simulink library "formationFlyingBlockset"  (R2015b)
settings: Solver=ode45  StartTime=0.0  StopTime=10.0  RelTol=1e-3
undefined symbols (not defined in the file): adaptive, aircraftmask_ID, aircraftmask_navigationLaw, aircraftmask_originNED_ECEF_rrm, aircraftmask_p0_NED_m, aircraftmask_phithetapsi0, aircraftmask_phithetapsi_trim, aircraftmask_pqr0, aircraftmask_uvw0, aircraftmask_wakevortexenabled, airkraftmask_displayLeader, DiscIntNeverNeededParam, Earth, fflib_degdegm2rrm, fflib_Hz2radps, fflib_rrm2degdegm, flat2lla, hinf, innerloop, Klqr, lquadr, mask_ac, mask_ID, mpc, outerloop, poleplacement, tatestos, uavsim, washout, WGS84
libraries: formationFlyingBlockset x59, aerolibtransform2 x42, simulink_extras x27, dspsrcs4 x11, aerolibutil x5, uavsimBlockset_ServoHS55 x4, uavsimBlockset_VectorNorm x3, uavsimBlockset_UAV3DVisualization x3, uavsimBlockset_AugmentWind x3, uavsimBlockset_UAV3DInterface x3, stringquartett x2, Parrot_DCAS_lib x2
(part 3 of 5)

== system formationFlyingBlockset/Attitude laws/Local rotation angle attitude control ==
  Plant : Inport  OutDataTypeStr=Bus: StateBus
  q_c : Inport  Port=2
  Attitude control Local rotation angles : Scope  NumInputPorts=2
  Bus Selector : BusSelector  OutputSignals=alpha_rad
  Bus Selector1 : BusSelector  OutputSignals=omega_b_rps
  "Compute local theta, phi, n_z" : Subsystem
  Ground1 : Ground
  Ground3 : Ground
  Hinf law theta - phi : Subsystem
  Mux : Mux
  Radians to Degrees{,1..3} (4 alike) : simulink_extras/Transformations/Radians to Degrees
  Remove operating point offset : Sum  Inputs=+-
  Scope : Scope
  Transfer Fcn : TransferFcn  Numerator=washout.num  Denominator=washout.den
  Trim AoA : Constant  Value=mask_ac.alpha_trim
  Yaw damper : Gain  Gain=uavsim.ap.control.yawdamper.K
  get r : Selector  InputPortWidth=3  IndexOptions=Index vector (dialog)  Indices=3  OutputSizes=1
  uHinf : Scope  NumInputPorts=2
  u : Outport
  wires:
  Transfer Fcn/1 -> Yaw damper/1
  get r/1 -> Transfer Fcn/1
  Bus Selector1/1 -> get r/1  "<omega_b_rps>"
  Remove operating point offset/1 -> Hinf law theta - phi/4(alpha_rad)
  Trim AoA/1 -> Remove operating point offset/2
  Bus Selector/1 -> Remove operating point offset/1  "<alpha_rad>"
  Mux/1 -> u/1
  q_c/1 -> "Compute local theta, phi, n_z"/2(q_c)
  Ground3/1 -> Hinf law theta - phi/3("theta_c, phi_c local")
  "Compute local theta, phi, n_z"/2("p, q") -> Hinf law theta - phi/2("p, q")
  "Compute local theta, phi, n_z"/1("theta, phi local") -> Hinf law theta - phi/1("theta, phi local")
  Plant/1 -> Bus Selector/1, Bus Selector1/1, "Compute local theta, phi, n_z"/1(Plant)
  Hinf law theta - phi/2(delta_e) -> Radians to Degrees3/1, Mux/2
  Radians to Degrees3/1 -> uHinf/2  "de_deg"
  Radians to Degrees2/1 -> uHinf/1  "da_deg"
  Radians to Degrees1/1 -> Attitude control Local rotation angles/2  "phi_deg"
  Radians to Degrees/1 -> Attitude control Local rotation angles/1  "theta_deg"
  Hinf law theta - phi/4(perf_phi) -> Radians to Degrees1/1
  Hinf law theta - phi/3(perf_theta) -> Radians to Degrees/1
  Hinf law theta - phi/1(delta_a) -> Mux/1, Radians to Degrees2/1
  Yaw damper/1 -> Mux/3, Scope/1
  Ground1/1 -> Mux/4

== system formationFlyingBlockset/Command laws - code generation -/LQR altitude ==
  State estimate : Inport
  Add1 : Sum  Inputs=+-
  Bus Selector2 : BusSelector  OutputSignals=p_ned_m,v_ned_mps
  Discrete-Time Integrator : DiscreteIntegrator  InitialConditionSetting=State (most efficient)  SampleTime=-1  ICPrevOutput=DiscIntNeverNeededParam  ICPrevScaledInput=DiscIntNeverNeededParam
  K LQR : Gain  Gain=lquadr.altitudeQuad.K  Multiplication=Matrix(K*u)
  Mux2 : Mux  Inputs=3
  Scope1 : Scope
  Selector : Selector  InputPortWidth=3  IndexOptions=Index vector (dialog)  Indices=3  OutputSizes=1
  Selector1 : Selector  InputPortWidth=3  IndexOptions=Index vector (dialog)  Indices=3  OutputSizes=1
  desired z_NED_m : Constant  Value=-1
  u : Outport
  wires:
  Selector/1 -> Add1/1  "z"
  Bus Selector2/1 -> Selector/1  "<p_ned_m>"
  Bus Selector2/2 -> Selector1/1  "<v_ned_mps>"
  Add1/1 -> Scope1/1, Mux2/1, Discrete-Time Integrator/1  "z"
  Selector1/1 -> Mux2/2  "vz"
  Discrete-Time Integrator/1 -> Mux2/3
  Mux2/1 -> K LQR/1
  K LQR/1 -> u/1
  desired z_NED_m/1 -> Add1/2
  State estimate/1 -> Bus Selector2/1

== system formationFlyingBlockset/Command laws - code generation -/LQR attitude ==
  State estimate : Inport
  Bus Selector1 : BusSelector  OutputSignals=quat_be,omega_b_rps
  Discrete-Time Integrator1 : DiscreteIntegrator  InitialConditionSetting=State (most efficient)  SampleTime=-1  ICPrevOutput=DiscIntNeverNeededParam  ICPrevScaledInput=DiscIntNeverNeededParam
  K LQR1 : Gain  Gain=lquadr.attitudeQuad.K  Multiplication=Matrix(K*u)
  Mux : Mux  Inputs=2
  Mux1 : Mux  Inputs=2
  Quaternions to Rotation Angles : aerolibtransform2/Quaternions to Rotation Angles  rotationOrder=ZYX
  Scope : Scope
  u : Outport
  wires:
  Quaternions to Rotation Angles/1 -> Mux/1, Discrete-Time Integrator1/1
  Mux/1 -> Mux1/1
  K LQR1/1 -> Scope/1, u/1
  Discrete-Time Integrator1/1 -> Mux1/2
  Mux1/1 -> K LQR1/1
  State estimate/1 -> Bus Selector1/1
  Bus Selector1/1 -> Quaternions to Rotation Angles/1  "<quat_be>"
  Bus Selector1/2 -> Mux/2  "<omega_b_rps>"

== system formationFlyingBlockset/Command laws - code generation -/LQR roll & pitch ==
  State estimate : Inport
  Bus Selector1 : BusSelector  OutputSignals=quat_be,omega_b_rps
  Discrete-Time Integrator1 : DiscreteIntegrator  InitialConditionSetting=State (most efficient)  SampleTime=-1  ICPrevOutput=DiscIntNeverNeededParam  ICPrevScaledInput=DiscIntNeverNeededParam
  K LQR1 : Gain  Gain=lquadr.rollpitchQuad.K  Multiplication=Matrix(K*u)
  Mux : Mux  Inputs=2
  Mux1 : Mux  Inputs=2
  Quaternions to Rotation Angles : aerolibtransform2/Quaternions to Rotation Angles  rotationOrder=ZYX
  "get p, q" : Selector  InputPortWidth=3  IndexOptions=Index vector (dialog)  Indices=[1 2]  OutputSizes=1
  "get theta, phi" : Selector  InputPortWidth=3  IndexOptions=Index vector (dialog)  Indices=[2 3]  OutputSizes=1
  u : Outport
  wires:
  Bus Selector1/2 -> "get p, q"/1  "<omega_b_rps>"
  Quaternions to Rotation Angles/1 -> "get theta, phi"/1
  Bus Selector1/1 -> Quaternions to Rotation Angles/1  "<quat_be>"
  "get p, q"/1 -> Mux/2
  State estimate/1 -> Bus Selector1/1
  Mux1/1 -> K LQR1/1
  Discrete-Time Integrator1/1 -> Mux1/2
  K LQR1/1 -> u/1
  Mux/1 -> Mux1/1
  "get theta, phi"/1 -> Discrete-Time Integrator1/1, Mux/1

== system formationFlyingBlockset/Cularis/Wake vortex effects ==
  AirframeBus : Inport  OutDataTypeStr=Bus: Airframe
  Environment : Inport  Port=2  OutDataTypeStr=Bus: Environment
  Ci_w : Inport  Port=3
  Augment atmospheric wind and wind gradients by induced wind and effects of induced wind gradients : uavsimBlockset_AugmentWind/Augment atmospheric wind and wind gradients by induced wind and induced wind gradients
  Constant : Constant  Value=aircraftmask_wakevortexenabled
  Constant1 : Constant  Value=zeros(3,1)
  Constant2 : Constant  Value=zeros(3,1)
  If : If  IfExpression=u1 ~= 0
  Subsystem : Subsystem
  Switch : Switch  Criteria=u2 ~= 0
  Switch1 : Switch  Criteria=u2 ~= 0
  Terminator : Terminator
  EnvData_augmented : Outport  OutDataTypeStr=Bus: Environment
  Vi_bfrozen : Outport  Port=2
  wires:
  AirframeBus/1 -> Subsystem/1(AirframeBus)
  Constant/1 -> Switch/2, Switch1/2, If/1
  Ci_w/1 -> Subsystem/2(Ci_w)
  Environment/1 -> Augment atmospheric wind and wind gradients by induced wind and effects of induced wind gradients/1
  Subsystem/1(Vi_bfrozen) -> Switch/1
  Subsystem/2(omegai_bfrozen) -> Switch1/1
  Constant1/1 -> Switch/3
  Switch/1 -> Vi_bfrozen/1, Augment atmospheric wind and wind gradients by induced wind and effects of induced wind gradients/2
  Switch1/1 -> Augment atmospheric wind and wind gradients by induced wind and effects of induced wind gradients/3
  Constant2/1 -> Switch1/3
  Augment atmospheric wind and wind gradients by induced wind and effects of induced wind gradients/1 -> EnvData_augmented/1
  If/1 -> Subsystem/Action
  If/2 -> Terminator/1

== system formationFlyingBlockset/Fixed wing avionics/Command laws ==
  Aircraft state estimate : Inport  OutDataTypeStr=Bus: StateBus
  iUASCom : Inport  Port=2  OutDataTypeStr=Bus: iUAScom
  formationOffset_m : Inport  Port=3
  fstate_dx_in : Inport  Port=4
  vLeaderState : Inport  Port=5  OutDataTypeStr=Bus: iUAScom
  Add1 : Sum
  Adds Separate Surface Excitations for system identification : Subsystem
  Constant : Constant  Value=100
  Constant1 : Constant  Value=aircraftmask_ID
  Constant2 : Constant  Value=airkraftmask_displayLeader
  Control laws : Subsystem  SystemSampleTime=uavsim.ap.hardware.dt_navigationloops_s
  If : If  IfExpression=u1 ~= 0  SampleTime=uavsim.ap.hardware.dt_navigationloops_s
  Leader NED position : formationFlyingBlockset/Signal to workspace  mask_id=['log_pNED_leader_UAS' num2str(aircraftmask_ID) ]  mask_dt=0.1  mask_debug=log_pNED_leader_UAS1
  Leader NED velocity : formationFlyingBlockset/Signal to workspace  mask_id=['log_vNED_leader_UAS' num2str(aircraftmask_ID) ]  mask_dt=0.1  mask_debug=log_vNED_leader_UAS1
  Scope : Scope
  Subsystem : Subsystem
  Terminator : Terminator
  u - system inputs : Outport  OutDataTypeStr=Bus: CMD
  fstate_dx : Outport  Port=2
  wires:
  Add1/1 -> Subsystem/1(In1)
  vLeaderState/1 -> Control laws/5(vLeaderState)
  Constant2/1 -> If/1
  If/1 -> Subsystem/Action
  If/2 -> Terminator/1
  Aircraft state estimate/1 -> Control laws/1(Plant)
  iUASCom/1 -> Control laws/2(iUASCom)
  formationOffset_m/1 -> Control laws/3(formationOffset_m)
  Constant1/1 -> Add1/1
  Constant/1 -> Add1/2
  Control laws/2(vc_NED_mps) -> Leader NED velocity/1, Subsystem/3(In3)
  Control laws/1(pc_NED_m) -> Scope/1, Leader NED position/1, Subsystem/2(In2)
  Adds Separate Surface Excitations for system identification/1(u + SSE) -> u - system inputs/1
  Control laws/3(CMD) -> Adds Separate Surface Excitations for system identification/1(u)
  Control laws/4(fstate_dx) -> fstate_dx/1
  fstate_dx_in/1 -> Control laws/4(fstate_dx_in)

== system formationFlyingBlockset/Fixed wing avionics/Sensor delays1 ==
  sensor readings : Inport  OutDataTypeStr=Bus: SensorBus
  Bus Creator : BusCreator  Inputs=7  OutDataTypeStr=Bus: SensorBus
  Bus Selector : BusSelector  OutputSignals=ahrs,airdata,gnss_l1,gnss_rtk,propulsion,radiodistance,windangles
  estimated aircraft state : Outport  OutDataTypeStr=Bus: StateBus
  wires:
  sensor readings/1 -> Bus Selector/1
  ? -> estimated aircraft state/1

== system formationFlyingBlockset/Parrot drone open loop dynamics/Vehicle model ==
  CMD : Inport  OutDataTypeStr=Bus: CMD_quadrotor
  EnvData : Inport  Port=2
  FM_external : Inport  Port=3
  Bus Selector2 : BusSelector  OutputSignals=groundlevel_NED_m,glocal_ms2
  Bus Selector3 : BusSelector  OutputSignals=RotationalVelocity.omega_b_rps,Velocity.Vground_bfrozen_mps,Attitude.euler_rad
  FIXME Remove algebraic loop : Memory  X0=1e-6
  Kinematics : uavsimblockset_SixDOFKinematics/Aircraft kinematics  mask_inertia=Itot  mask_mass=mtot  mask_P0_ECEF_rrm=mask_p0_ECEF_lla  mask_originNED_ECEF_rrm=mask_originNED_ECEF_rrm  mask_uvw0=mask_uvw0  mask_phithetapsi0=mask_phithetapsi0  mask_omega0=mask_pqr0
  ModelBus6 : BusCreator  Inputs=2  OutDataTypeStr=Bus: Airframe  NonVirtualBus=on
  Parrot dynamics : Subsystem
  Airframe : Outport  OutDataTypeStr=Bus: Airframe
  Cwind : Outport  Port=2
  FMprop : Outport  Port=3
  wires:
  FIXME Remove algebraic loop/1 -> ModelBus6/1, Bus Selector3/1  "Kinematics"
  Bus Selector2/1 -> Kinematics/1  "<groundlevel_NED_m>"
  Bus Selector2/2 -> Kinematics/4  "<glocal_ms2>"
  Bus Selector3/1 -> Parrot dynamics/3(omega_bfrozen_rps)  "<omega_b_rps>"
  Bus Selector3/2 -> Parrot dynamics/4(Vground_bfrozen_mps)  "<Vground_bfrozen_mps>"
  ModelBus6/1 -> Airframe/1
  Parrot dynamics/2(AeroBus) -> ModelBus6/2
  EnvData/1 -> Bus Selector2/1, Parrot dynamics/2(EnvData)
  FM_external/1 -> Kinematics/3
  Parrot dynamics/3(Coefficients_windframe) -> Cwind/1
  Parrot dynamics/1(FMaero_bf) -> Kinematics/2
  Kinematics/1 -> FIXME Remove algebraic loop/1
  CMD/1 -> Parrot dynamics/1(CMD)
  Bus Selector3/3 -> Parrot dynamics/5(eulers)  "<euler_rad>"

== system formationFlyingBlockset/Quadcopter avionics/Command laws - code generation - ==
  Aircraft state estimate : Inport  OutDataTypeStr=Bus: StateBus
  Control laws : Subsystem  TreatAsAtomicUnit=on  SystemSampleTime=uavsim.ap.hardware.dt_attitudeloops_s
  u - system inputs : Outport  OutDataTypeStr=Bus: CMD
  wires:
  Control laws/1(engine commands) -> u - system inputs/1
  Aircraft state estimate/1 -> Control laws/1(Plant state estimate)

== system formationFlyingBlockset/Quadcopter avionics/Sensor delays1 ==
  sensor readings : Inport  OutDataTypeStr=Bus: SensorBus
  Bus Creator : BusCreator  Inputs=7  OutDataTypeStr=Bus: SensorBus
  Bus Selector : BusSelector  OutputSignals=ahrs,airdata,gnss_l1,gnss_rtk,propulsion,radiodistance,windangles
  estimated aircraft state : Outport  OutDataTypeStr=Bus: StateBus
  wires:
  ? -> estimated aircraft state/1
  sensor readings/1 -> Bus Selector/1

== system formationFlyingBlockset/Sensor package: error-free/AHRS ==
  aircraft state : Inport  OutDataTypeStr=Bus: Airframe
  Environment : Inport  Port=2  OutDataTypeStr=Bus: Environment
  Add gravity : Sum
  Bus Creator : BusCreator  Inputs=3  OutDataTypeStr=Bus: AHRS
  Bus Selector : BusSelector  OutputSignals=Kinematics.Attitude.DCM_be,Kinematics.RotationalVelocity.omega_b_rps,Kinematics.Acceleration.VgroundDot_bfrozen_mps2,Kinematics.RotationalAcceleration.omegaDot_b_rps2
  Bus Selector1 : BusSelector  OutputSignals=glocal_ms2
  Constant : Constant  Value=[0 0 0]'
  Constant1 : Constant  Value=[0 0]'
  Direction Cosine Matrix to Quaternions : aerolibtransform2/Direction Cosine Matrix  to Quaternions
  Mux : Mux  Inputs=2
  Mux2 : Mux  Inputs=2
  Scope1 : Scope
  Three-axis Accelerometer : aerolibnav/Three-axis Accelerometer  units=Metric (MKS)  acc=[0 0 0]  gtype=off  dtype_a=off  w_a=190  z_a=0.707  a_sf_cc=[1 0 0; 0 1 0; 0 0 1]  a_bias=[0 0 0]  a_Ts=0.01  a_rand=off  a_seeds=[23093 23094 23095]  a_pow=0.01 * [0.0101 0.0116 0.0144] .^ 2  a_sat="[-inf  -inf  -inf  inf inf inf]"
  Three-axis Gyroscope : aerolibnav/Three-axis Gyroscope  dtype_g=off  w_g=190  z_g=0.707  g_sf_cc=[1 0 0; 0 1 0; 0 0 1]  g_bias=[0 0 0]  g_sen=[0 0 0]  g_Ts=0.01  g_rand=off  g_seeds=[23093 23094 23095]  g_pow="0.01 * (1e-3 * [0.8056    0.5346    0.9000]) .^2"  g_sat="[-inf  -inf  -inf  inf inf inf]"
  gravity to body frame : Product  Multiplication=Matrix(*)
  unit conversion: mps2 to g : formationFlyingBlockset/unit conversion: mps2 to g
  output : Outport  OutDataTypeStr=Bus: AHRS
  wires:
  Mux2/1 -> Scope1/1
  Bus Creator/1 -> output/1
  aircraft state/1 -> Bus Selector/1
  Bus Selector/1 -> Direction Cosine Matrix to Quaternions/1, gravity to body frame/1  "<DCM_be>"
  Direction Cosine Matrix to Quaternions/1 -> Bus Creator/1  "quat"
  Bus Selector/2 -> Three-axis Gyroscope/1, Three-axis Accelerometer/2  "<omega_b_rps>"
  Bus Selector/3 -> Add gravity/1  "<VgroundDot_bfrozen_mps2>"
  Three-axis Gyroscope/1 -> Bus Creator/2  "gyro_rps"
  Three-axis Accelerometer/1 -> Bus Creator/3, Mux2/1  "acc_mps2"
  Bus Selector/4 -> Three-axis Accelerometer/3  "<omegaDot_b_rps2>"
  Constant/1 -> Three-axis Accelerometer/4
  Bus Selector1/1 -> Mux/2  "<glocal_ms2>"
  Environment/1 -> Bus Selector1/1
  gravity to body frame/1 -> Add gravity/2
  Constant1/1 -> Mux/1
  Mux/1 -> gravity to body frame/2
  Add gravity/1 -> unit conversion: mps2 to g/1, Three-axis Accelerometer/1, Mux2/2
  unit conversion: mps2 to g/1 -> Three-axis Gyroscope/2

== system formationFlyingBlockset/Sensor package: error-free/Air Data ==
  aircraft state : Inport  OutDataTypeStr=Bus: Airframe
  Bus Creator : BusCreator  Inputs=3  OutDataTypeStr=Bus: Airdata
  Bus Selector : BusSelector  OutputSignals=Kinematics.Position.P_LLA_deg_m,Aero.qbar_Pa
  Gain : Gain
  ISA Atmosphere Model : aerolibatmos2/ISA Atmosphere Model  custom=off  g=9.80665  gamma=1.4  R=287.0531  L=0.0065  h_trop=11000  h_strat=20000  rho0=1.225  P0=101325  T0=288.15  h0=0
  Terminator : Terminator
  Terminator1 : Terminator
  get altitude : Selector  InputPortWidth=3  IndexOptions=Index vector (dialog)  Indices=3  OutputSizes=1
  output : Outport  OutDataTypeStr=Bus: Airdata
  wires:
  get altitude/1 -> ISA Atmosphere Model/1
  Gain/1 -> Bus Creator/3  "qBar_Pa"
  ISA Atmosphere Model/4 -> Terminator1/1
  ISA Atmosphere Model/2 -> Terminator/1
  ISA Atmosphere Model/3 -> Bus Creator/2  "pStat_Pa"
  ISA Atmosphere Model/1 -> Bus Creator/1  "Tair_K"
  Bus Selector/1 -> get altitude/1  "<P_LLA_deg_m>"
  Bus Selector/2 -> Gain/1  "<qbar_Pa>"
  Bus Creator/1 -> output/1
  aircraft state/1 -> Bus Selector/1

== system formationFlyingBlockset/Sensor package: error-free/L1 GPS ==
  aircraft state : Inport  OutDataTypeStr=Bus: Airframe
  Bus Creator : BusCreator  Inputs=2  OutDataTypeStr=Bus: GNSSL1
      settings: InheritFromInputs=off
  Bus Selector1 : BusSelector  OutputSignals=Kinematics.Position.P_ECEF_m,Kinematics.Velocity.Vground_ECEF_mps
  Gain : Gain
  Gain1 : Gain
  output : Outport  OutDataTypeStr=Bus: GNSSL1
  wires:
  Gain1/1 -> Bus Creator/2  "v_ecef_m"
  Gain/1 -> Bus Creator/1  "p_ecef_m"
  Bus Selector1/2 -> Gain1/1  "<Vground_ECEF_mps>"
  Bus Selector1/1 -> Gain/1  "<P_ECEF_m>"
  Bus Creator/1 -> output/1
  aircraft state/1 -> Bus Selector1/1

== system formationFlyingBlockset/Sensor package: error-free/Optitrack ==
  aircraft state : Inport  OutDataTypeStr=Bus: Airframe
  Bus Creator : BusCreator  Inputs=2  OutDataTypeStr=Bus: MotionTracker
      settings: InheritFromInputs=off
  Bus Selector : BusSelector  OutputSignals=Kinematics.Position.P_NED_m,Kinematics.Velocity.Vground_NED_mps
  Gain : Gain
  Gain1 : Gain
  output : Outport  OutDataTypeStr=Bus: MotionTracker
  wires:
  Bus Creator/1 -> output/1
  aircraft state/1 -> Bus Selector/1
  Bus Selector/1 -> Gain/1  "<P_NED_m>"
  Gain/1 -> Bus Creator/1  "p_ned_m"
  Bus Selector/2 -> Gain1/1  "<Vground_NED_mps>"
  Gain1/1 -> Bus Creator/2  "v_ned_mps"

== system formationFlyingBlockset/Sensor package: error-free/Propulsion sensors ==
  aircraft state : Inport  OutDataTypeStr=Bus: Airframe
  Bus Creator : BusCreator  Inputs=2  OutDataTypeStr=Bus: Enginedata
      settings: InheritFromInputs=off
  I : Constant  Value=0
  U : Constant  Value=0
  output : Outport  OutDataTypeStr=Bus: Enginedata
  wires:
  Bus Creator/1 -> output/1
  I/1 -> Bus Creator/2  "I"
  U/1 -> Bus Creator/1  "U"

== system formationFlyingBlockset/Sensor package: error-free/RTK DGPS ==
  aircraft state : Inport  OutDataTypeStr=Bus: Airframe
  inter UAS com : Inport  Port=2  OutDataTypeStr=Bus: iUAScom
  Bus Creator : BusCreator  Inputs=2  OutDataTypeStr=Bus: GNSSRTK
      settings: InheritFromInputs=off
  Bus Selector : BusSelector  OutputSignals=P_NED_m,Vground_NED_mps
  Bus Selector1 : BusSelector  OutputSignals=Kinematics.Position.P_NED_m,Kinematics.Velocity.Vground_NED_mps
  Delta position : Sum  Inputs=+-
  Delta velocity : Sum  Inputs=+-
  Flat Earth to LLA{,2..4} (4 alike) : aerolibtransform2/Flat Earth to LLA  units=Metric (MKS)  ptype=Earth (WGS84)  F=1/298.257223563  R=6378137  LL0=rad2deg(aircraftmask_originNED_ECEF_rrm(1:2))  psi=0
  LLA to ECEF Position{,2..4} (4 alike) : aerolibtransform2/LLA to ECEF Position  units=Metric (MKS)  ptype=Earth (WGS84)  F=1/298.257223563  R=6378137
  Scope : Scope
  Scope1 : Scope
  Scope2 : Scope
  href NED : Constant  Value=aircraftmask_originNED_ECEF_rrm(3)
  output : Outport  OutDataTypeStr=Bus: GNSSRTK
  wires:
  Delta velocity/1 -> Bus Creator/2  "delta_v_ecef_mps"
  LLA to ECEF Position3/1 -> Delta velocity/1
  LLA to ECEF Position4/1 -> Delta velocity/2
  Flat Earth to LLA4/1 -> LLA to ECEF Position4/1
  Flat Earth to LLA4/2 -> LLA to ECEF Position4/2
  Bus Selector/2 -> Flat Earth to LLA4/1  "<Vground_NED_mps>"
  Flat Earth to LLA3/1 -> LLA to ECEF Position3/1
  Flat Earth to LLA3/2 -> LLA to ECEF Position3/2
  href NED/1 -> Flat Earth to LLA/2, Flat Earth to LLA2/2, Flat Earth to LLA4/2, Flat Earth to LLA3/2
  Bus Selector1/2 -> Flat Earth to LLA3/1  "<Vground_NED_mps>"
  LLA to ECEF Position/1 -> Delta position/1
  LLA to ECEF Position2/1 -> Delta position/2
  Flat Earth to LLA2/1 -> LLA to ECEF Position2/1
  Flat Earth to LLA2/2 -> LLA to ECEF Position2/2
  Delta position/1 -> Bus Creator/1, Scope/1  "delta_p_ecef_m"
  Bus Selector/1 -> Scope2/1, Flat Earth to LLA2/1  "<P_NED_m>"
  Flat Earth to LLA/1 -> LLA to ECEF Position/1
  Flat Earth to LLA/2 -> LLA to ECEF Position/2
  Bus Selector1/1 -> Scope1/1, Flat Earth to LLA/1  "<P_NED_m>"
  Bus Creator/1 -> output/1
  aircraft state/1 -> Bus Selector1/1
  inter UAS com/1 -> Bus Selector/1

== system formationFlyingBlockset/Sensor package: error-free/Radio distance sensor ==
  aircraft state : Inport  OutDataTypeStr=Bus: Airframe
  inter UAS com : Inport  Port=2  OutDataTypeStr=Bus: iUAScom
  Bus Creator : BusCreator  Inputs=1  OutDataTypeStr=Bus: Radiodistance
      settings: InheritFromInputs=off
  Bus Selector : BusSelector  OutputSignals=P_NED_m
  Bus Selector1 : BusSelector  OutputSignals=Kinematics.Position.P_NED_m
  Delta position : Sum  Inputs=-+
  vector norm : uavsimBlockset_VectorNorm/vector norm
  output : Outport  OutDataTypeStr=Bus: Radiodistance
  wires:
  vector norm/1 -> Bus Creator/1  "r"
  Delta position/1 -> vector norm/1
  Bus Creator/1 -> output/1
  Bus Selector/1 -> Delta position/2  "<P_NED_m>"
  Bus Selector1/1 -> Delta position/1  "<P_NED_m>"
  aircraft state/1 -> Bus Selector1/1
  inter UAS com/1 -> Bus Selector/1

== system formationFlyingBlockset/Sensor package: error-free/Wind angle sensors ==
  aircraft state : Inport  OutDataTypeStr=Bus: Airframe
  Bus Creator : BusCreator  Inputs=2  OutDataTypeStr=Bus: WindAngles
  Bus Selector : BusSelector  OutputSignals=Aero.alpha_rad,Aero.beta_rad
  Gain : Gain
  Gain1 : Gain
  output : Outport  OutDataTypeStr=Bus: WindAngles
  wires:
  Gain1/1 -> Bus Creator/2  "beta_rad"
  Gain/1 -> Bus Creator/1  "alpha_rad"
  Bus Selector/2 -> Gain1/1  "<beta_rad>"
  Bus Selector/1 -> Gain/1  "<alpha_rad>"
  aircraft state/1 -> Bus Selector/1
  Bus Creator/1 -> output/1

== system formationFlyingBlockset/Wake vortex effects/Subsystem ==
  AirframeBus : Inport  OutDataTypeStr=Bus: Airframe
  Ci_w : Inport  Port=2
  Action Port : ActionPort
  Bus Selector : BusSelector  OutputSignals=Kinematics.Position.P_NED_m,Kinematics.Velocity.Vground_NED_mps,Kinematics.Attitude.DCM_be,Aero.alpha_rad,Aero.beta_rad
  Cularis Vortex model : formationFlyingBlockset/Cularis Vortex model  mask_ID=aircraftmask_ID
  Demux : Demux  Outputs=2
  Direction Cosine Matrix  to Quaternions : aerolibtransform2/Direction Cosine Matrix  to Quaternions
  Get CL : Selector  InputPortWidth=6  IndexOptions=Index vector (dialog)  Indices=3  OutputSizes=1
  Memory : Memory  X0=[0 0]
  Memory1 : Memory  X0=eye(3)
  Memory2 : Memory  X0=zeros(3,1)
  Memory3 : Memory  X0=zeros(3,1)
  Memory4 : Memory  X0=1
  Mux : Mux  Inputs=2
  Signal Conversion : SignalConversion
  Vi_bfrozen : Outport
  omegai_bfrozen : Outport  Port=2
  vortex parameters : Outport  Port=3
  wires:
  Demux/1 -> Cularis Vortex model/5
  Demux/2 -> Cularis Vortex model/6
  AirframeBus/1 -> Bus Selector/1
  Ci_w/1 -> Get CL/1
  Get CL/1 -> Memory4/1
  Direction Cosine Matrix  to Quaternions/1 -> Cularis Vortex model/4
  Bus Selector/1 -> Memory3/1  "<P_NED_m>"
  Bus Selector/2 -> Memory2/1  "<Vground_NED_mps>"
  Bus Selector/3 -> Memory1/1  "<DCM_be>"
  Bus Selector/4 -> Mux/1  "<alpha_rad>"
  Bus Selector/5 -> Mux/2  "<beta_rad>"
  Mux/1 -> Memory/1
  Memory/1 -> Demux/1
  Memory1/1 -> Direction Cosine Matrix  to Quaternions/1
  Memory2/1 -> Cularis Vortex model/2
  Memory3/1 -> Cularis Vortex model/1
  Memory4/1 -> Cularis Vortex model/3
  Cularis Vortex model/1 -> Vi_bfrozen/1
  Cularis Vortex model/2 -> omegai_bfrozen/1
  Cularis Vortex model/4 -> Signal Conversion/1
  Signal Conversion/1 -> vortex parameters/1

== system formationFlyingBlockset/Wake vortex effects/Visualize vortices in UAV3D ==
  vortex parameters : Inport
  enable UAV3D : Inport  Port=2
  Bus Selector : BusSelector  OutputSignals=p0_filament_left,p0_filament_right,dcm_ew
  Constant1 : Constant  Value=aircraftmask_ID+30
  Constant11 : Constant  Value=0.5
  Constant12 : Constant  Value=3*uavsim.cularis.b
  Constant13 : Constant  Value=0.3
  Constant2 : Constant  Value=aircraftmask_ID+60
  Display : Display
  Visualize vortex tunnel in UAV3D1 : formationFlyingBlockset/Visualize vortex tunnel in UAV3D
  Visualize vortex tunnel in UAV3D2 : formationFlyingBlockset/Visualize vortex tunnel in UAV3D
  wires:
  Bus Selector/2 -> Visualize vortex tunnel in UAV3D1/2  "<p0_filament_right>"
  Constant12/1 -> Visualize vortex tunnel in UAV3D1/4, Visualize vortex tunnel in UAV3D2/4
  Constant11/1 -> Visualize vortex tunnel in UAV3D1/3, Visualize vortex tunnel in UAV3D2/3
  Constant2/1 -> Visualize vortex tunnel in UAV3D2/1
  Bus Selector/1 -> Visualize vortex tunnel in UAV3D2/2, Display/1  "<p0_filament_left>"
  Constant1/1 -> Visualize vortex tunnel in UAV3D1/1
  Constant13/1 -> Visualize vortex tunnel in UAV3D1/5, Visualize vortex tunnel in UAV3D2/5
  vortex parameters/1 -> Bus Selector/1
  Bus Selector/3 -> Visualize vortex tunnel in UAV3D1/6, Visualize vortex tunnel in UAV3D2/6  "<dcm_ew>"
  enable UAV3D/1 -> Visualize vortex tunnel in UAV3D1/7, Visualize vortex tunnel in UAV3D2/7

== system formationFlyingBlockset/Zagi/Wake vortex effects ==
  AirframeBus : Inport  OutDataTypeStr=Bus: Airframe
  Environment : Inport  Port=2  OutDataTypeStr=Bus: Environment
  Ci_w : Inport  Port=3
  Augment atmospheric wind and wind gradients by induced wind and effects of induced wind gradients : uavsimBlockset_AugmentWind/Augment atmospheric wind and wind gradients by induced wind and induced wind gradients
  Constant : Constant  Value=aircraftmask_wakevortexenabled
  Constant1 : Constant  Value=zeros(3,1)
  Constant2 : Constant  Value=zeros(3,1)
  If : If  IfExpression=u1 ~= 0
  Subsystem : Subsystem
  Switch : Switch  Criteria=u2 ~= 0
  Switch1 : Switch  Criteria=u2 ~= 0
  Terminator : Terminator
  EnvData_augmented : Outport  OutDataTypeStr=Bus: Environment
  Vi_bfrozen : Outport  Port=2
  wires:
  AirframeBus/1 -> Subsystem/1(AirframeBus)
  Constant/1 -> Switch/2, Switch1/2, If/1
  Ci_w/1 -> Subsystem/2(Ci_w)
  Environment/1 -> Augment atmospheric wind and wind gradients by induced wind and effects of induced wind gradients/1
  Subsystem/1(Vi_bfrozen) -> Switch/1
  Subsystem/2(omegai_bfrozen) -> Switch1/1
  Constant1/1 -> Switch/3
  Switch/1 -> Vi_bfrozen/1, Augment atmospheric wind and wind gradients by induced wind and effects of induced wind gradients/2
  Switch1/1 -> Augment atmospheric wind and wind gradients by induced wind and effects of induced wind gradients/3
  Constant2/1 -> Switch1/3
  Augment atmospheric wind and wind gradients by induced wind and effects of induced wind gradients/1 -> EnvData_augmented/1
  If/1 -> Subsystem/Action
  If/2 -> Terminator/1

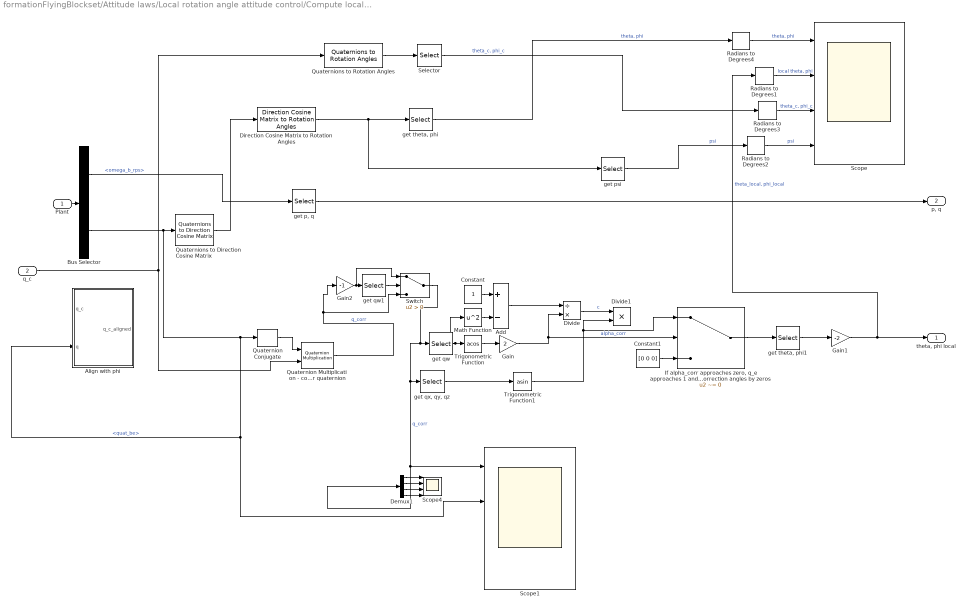
== system formationFlyingBlockset/Attitude laws/Local rotation angle attitude control/Compute local theta, phi, n_z ==
  Plant : Inport  OutDataTypeStr=Bus: StateBus
  q_c : Inport  Port=2
  Add : Sum  Inputs=+-
  Align with phi : Subsystem
  Bus Selector : BusSelector  OutputSignals=omega_b_rps,quat_be
  Constant : Constant
  Constant1 : Constant  Value=[0 0 0]
  Demux1 : Demux
  Direction Cosine Matrix to Rotation Angles : aerolibtransform2/Direction Cosine Matrix to Rotation Angles  rotationOrder=ZYX  lim=Default
      settings: AttributesFormatString=Rotation Order: %<rotationOrder>
  Divide : Product  Inputs=/*
  Divide1 : Product  Inputs=**
  Gain : Gain  Gain=2
  Gain1 : Gain  Gain=-2
  Gain2 : Gain  Gain=-1
  "If alpha_corr approaches zero, q_e approaches 1 and c goes to infinity. In that case, just replace the computed correction angles by zeros" : Switch  Criteria=u2 ~= 0
  Math Function : Math  Operator=square  SaturateOnIntegerOverflow=on
  Quaternion Conjugate : aerolibutil/Quaternion Conjugate
  Quaternion Multiplication - compute error quaternion : aerolibutil/Quaternion Multiplication
  Quaternions to Direction Cosine Matrix : aerolibtransform2/Quaternions to  Direction Cosine Matrix
  Quaternions to Rotation Angles : aerolibtransform2/Quaternions to Rotation Angles  rotationOrder=ZYX
  Radians to Degrees{1..4} (4 alike) : simulink_extras/Transformations/Radians to Degrees
  Scope : Scope  NumInputPorts=4
  Scope1 : Scope  NumInputPorts=4
  Scope4 : Scope  NumInputPorts=4
  Selector : Selector  InputPortWidth=3  IndexOptions=Index vector (dialog)  Indices=[2 3]  OutputSizes=1
  Switch : Switch  Criteria=u2 > Threshold
  Trigonometric Function : Trigonometry  Operator=acos
  Trigonometric Function1 : Trigonometry  Operator=asin
  "get p, q" : Selector  InputPortWidth=3  IndexOptions=Index vector (dialog)  Indices=[1 2]  OutputSizes=1
  get psi : Selector  InputPortWidth=3  IndexOptions=Index vector (dialog)  Indices=1  OutputSizes=1
  get qw : Selector  InputPortWidth=4  IndexOptions=Index vector (dialog)  Indices=1  OutputSizes=1
  get qw1 : Selector  InputPortWidth=4  IndexOptions=Index vector (dialog)  Indices=1  OutputSizes=1
  "get qx, qy, qz" : Selector  InputPortWidth=4  IndexOptions=Index vector (dialog)  Indices=2:4  OutputSizes=1
  "get theta, phi" : Selector  InputPortWidth=3  IndexOptions=Index vector (dialog)  Indices=[2 3]  OutputSizes=1
  "get theta, phi1" : Selector  InputPortWidth=3  IndexOptions=Index vector (dialog)  Indices=[2 1]  OutputSizes=1
  "theta, phi local" : Outport
  "p, q" : Outport  Port=2
  wires:
  get qw1/1 -> Switch/2
  Gain2/1 -> get qw1/1, Switch/1
  Quaternion Multiplication - compute error quaternion/1 -> Switch/3, Gain2/1  "q_corr"
  Demux1/1 -> Scope4/1
  Demux1/2 -> Scope4/2
  Demux1/4 -> Scope4/4
  Demux1/3 -> Scope4/3
  Radians to Degrees1/1 -> Scope/2  "local theta, phi"
  Radians to Degrees2/1 -> Scope/4  "psi"
  Radians to Degrees3/1 -> Scope/3  "theta_c, phi_c"
  Radians to Degrees4/1 -> Scope/1  "theta, phi"
  get psi/1 -> Radians to Degrees2/1  "psi"
  Selector/1 -> Radians to Degrees3/1  "theta_c, phi_c"
  Quaternions to Rotation Angles/1 -> Selector/1
  Gain1/1 -> "theta, phi local"/1, Radians to Degrees1/1  "theta_local, phi_local"
  Quaternion Conjugate/1 -> Quaternion Multiplication - compute error quaternion/1
  "get theta, phi"/1 -> Radians to Degrees4/1  "theta, phi"
  "get theta, phi1"/1 -> Gain1/1
  "If alpha_corr approaches zero, q_e approaches 1 and c goes to infinity. In that case, just replace the computed correction angles by zeros"/1 -> "get theta, phi1"/1
  Constant1/1 -> "If alpha_corr approaches zero, q_e approaches 1 and c goes to infinity. In that case, just replace the computed correction angles by zeros"/3
  Trigonometric Function1/1 -> Divide1/2, "If alpha_corr approaches zero, q_e approaches 1 and c goes to infinity. In that case, just replace the computed correction angles by zeros"/1
  "get qx, qy, qz"/1 -> Trigonometric Function1/1
  Divide/1 -> Divide1/1  "c"
  Add/1 -> Divide/1
  Math Function/1 -> Add/2
  Constant/1 -> Add/1
  Gain/1 -> "If alpha_corr approaches zero, q_e approaches 1 and c goes to infinity. In that case, just replace the computed correction angles by zeros"/2, Divide/2  "alpha_corr"
  Trigonometric Function/1 -> Gain/1
  get qw/1 -> Trigonometric Function/1, Math Function/1
  Switch/1 -> get qw/1, "get qx, qy, qz"/1, Scope1/1, Demux1/1  "q_corr"
  q_c/1 -> Quaternion Multiplication - compute error quaternion/2, Quaternions to Rotation Angles/1
  Quaternions to Direction Cosine Matrix/1 -> Direction Cosine Matrix to Rotation Angles/1
  Bus Selector/2 -> Quaternion Conjugate/1, Align with phi/2(q), Scope1/2, Quaternions to Direction Cosine Matrix/1  "<quat_be>"
  "get p, q"/1 -> "p, q"/1
  Direction Cosine Matrix to Rotation Angles/1 -> "get theta, phi"/1, get psi/1
  Bus Selector/1 -> "get p, q"/1  "<omega_b_rps>"
  Plant/1 -> Bus Selector/1

== system formationFlyingBlockset/Attitude laws/Local rotation angle attitude control/Hinf law theta - phi ==
  "theta, phi local" : Inport
  "p, q" : Inport  Port=2
  "theta_c, phi_c local" : Inport  Port=3
  alpha_rad : Inport  Port=4
  C PD : Subsystem
  Demux : Demux  Outputs=2
  Mux1 : Mux  Inputs=2
  get phis : Selector  InputPortWidth=4  IndexOptions=Index vector (dialog)  Indices=[2 4]  OutputSizes=1
  get thetas : Selector  InputPortWidth=4  IndexOptions=Index vector (dialog)  Indices=[1 3]  OutputSizes=1
  delta_a : Outport
  delta_e : Outport  Port=2
  perf_theta : Outport  Port=3
  perf_phi : Outport  Port=4
  wires:
  alpha_rad/1 -> C PD/4(alpha_rad)
  "theta_c, phi_c local"/1 -> Mux1/2, C PD/2(eulers_c)
  "theta, phi local"/1 -> Mux1/1, C PD/1(eulers)
  get phis/1 -> perf_phi/1
  get thetas/1 -> perf_theta/1
  Mux1/1 -> get thetas/1, get phis/1
  "p, q"/1 -> C PD/3(p,q)
  Demux/2 -> delta_e/1
  Demux/1 -> delta_a/1
  C PD/1("da, de") -> Demux/1

== system formationFlyingBlockset/Cularis/Wake vortex effects/Subsystem ==
  AirframeBus : Inport  OutDataTypeStr=Bus: Airframe
  Ci_w : Inport  Port=2
  Action Port : ActionPort
  Aerodynamic interaction interface : formationFlyingBlockset/Aerodynamic interaction interface  mask_c_m=uavsim.cularis.c  mask_ID=aircraftmask_ID  mask_wingspan_m=uavsim.cularis.b  mask_sweepangle_rad=uavsim.cularis.wingsweep_rad  mask_dihedral_rad=uavsim.cularis.dihedral_rad  mask_l_longi_m=uavsim.cularis.c  mask_nosecoo_m=[uavsim.cularis.c/2 0 0]  mask_l_vertical_m=0.05  mask_fincoo_m=[0 0 -0.05]
  Bus Selector : BusSelector  OutputSignals=Kinematics.Position.P_NED_m,Kinematics.Velocity.Vground_NED_mps,Kinematics.Attitude.DCM_be,Aero.alpha_rad,Aero.beta_rad
  Direction Cosine Matrix  to Quaternions : aerolibtransform2/Direction Cosine Matrix  to Quaternions
  Get CL : Selector  InputPortWidth=6  IndexOptions=Index vector (dialog)  Indices=3  OutputSizes=1
  Memory : Memory  X0=[0 0]
  Memory1 : Memory  X0=eye(3)
  Memory2 : Memory  X0=zeros(3,1)
  Memory3 : Memory  X0=zeros(3,1)
  Memory4 : Memory  X0=1
  Mux : Mux  Inputs=2
  Terminator : Terminator
  Vi_bfrozen : Outport
  omegai_bfrozen : Outport  Port=2
  wires:
  AirframeBus/1 -> Bus Selector/1
  Ci_w/1 -> Get CL/1
  Get CL/1 -> Memory4/1
  Direction Cosine Matrix  to Quaternions/1 -> Aerodynamic interaction interface/4
  Bus Selector/1 -> Memory3/1  "<P_NED_m>"
  Bus Selector/2 -> Memory2/1  "<Vground_NED_mps>"
  Bus Selector/3 -> Memory1/1  "<DCM_be>"
  Bus Selector/4 -> Mux/1  "<alpha_rad>"
  Bus Selector/5 -> Mux/2  "<beta_rad>"
  Mux/1 -> Memory/1
  Memory/1 -> Aerodynamic interaction interface/5
  Memory1/1 -> Direction Cosine Matrix  to Quaternions/1
  Memory2/1 -> Aerodynamic interaction interface/2
  Memory3/1 -> Aerodynamic interaction interface/1
  Memory4/1 -> Aerodynamic interaction interface/3
  Aerodynamic interaction interface/2 -> omegai_bfrozen/1
  Aerodynamic interaction interface/1 -> Vi_bfrozen/1
  Aerodynamic interaction interface/3 -> Terminator/1

== system formationFlyingBlockset/Fixed wing avionics/Command laws/Adds Separate Surface Excitations for system identification ==
  u : Inport  OutDataTypeStr=Bus: CMD
  "Add excitation signals to controller outputs " : Sum
  Bus Creator : BusCreator  Inputs=5  OutDataTypeStr=Bus: CMD  NonVirtualBus=on
      settings: InheritFromInputs=off
  Bus Selector : BusSelector  OutputSignals=da_rad,de_rad,dr_rad,den_0to1,df_rad
  Chirp Signal1 : simulink/Sources/Chirp Signal  f1=1  T=10  f2=5
  Constant{,1..3} (4 alike) : Constant  Value=0
  Demux : Demux  Outputs=5
  Gain : Gain  Gain=deg2rad(0)
  Mux : Mux  Inputs=5
  Mux1 : Mux  Inputs=5
  u + SSE : Outport  OutDataTypeStr=Bus: CMD
  wires:
  Bus Creator/1 -> u + SSE/1
  u/1 -> Bus Selector/1
  Constant1/1 -> Mux/3  "dr_rad"
  Constant/1 -> Mux/1  "da_rad"
  Constant3/1 -> Mux/5  "df_rad"
  Constant2/1 -> Mux/4  "den_0to1"
  Chirp Signal1/1 -> Gain/1
  Mux/1 -> "Add excitation signals to controller outputs "/1
  Mux1/1 -> "Add excitation signals to controller outputs "/2
  "Add excitation signals to controller outputs "/1 -> Demux/1
  Demux/2 -> Bus Creator/2  "de_rad"
  Demux/1 -> Bus Creator/1  "da_rad"
  Demux/3 -> Bus Creator/3  "dr_rad"
  Demux/4 -> Bus Creator/4  "den_0to1"
  Demux/5 -> Bus Creator/5  "df_rad"
  Bus Selector/2 -> Mux1/2  "<de_rad>"
  Bus Selector/1 -> Mux1/1  "<da_rad>"
  Bus Selector/3 -> Mux1/3  "<dr_rad>"
  Bus Selector/4 -> Mux1/4  "<den_0to1>"
  Bus Selector/5 -> Mux1/5  "<df_rad>"
  Gain/1 -> Mux/2  "de_rad"

== system formationFlyingBlockset/Fixed wing avionics/Command laws/Control laws ==
  Plant : Inport  OutDataTypeStr=Bus: StateBus
  iUASCom : Inport  Port=2  OutDataTypeStr=Bus: iUAScom
  formationOffset_m : Inport  Port=3
  fstate_dx_in : Inport  Port=4
  vLeaderState : Inport  Port=5  OutDataTypeStr=Bus: iUAScom
  Launch law -1 : Subsystem
  Multiport Switch : MultiPortSwitch  Inputs=4
  Navigation supervisor : Subsystem
  Test signal generator - 3 : Subsystem
  Trajectory law - 2 : Subsystem
  Trim inputs - 4 : Subsystem
  pc_NED_m : Outport
  vc_NED_mps : Outport  Port=2
  CMD : Outport  Port=3  OutDataTypeStr=Bus: CMD
  fstate_dx : Outport  Port=4
  wires:
  vLeaderState/1 -> Trajectory law - 2/6(vLeaderState)
  Trajectory law - 2/3(CMD) -> Multiport Switch/3
  Launch law -1/1(CMD) -> Multiport Switch/2
  Navigation supervisor/1(Active law index) -> Multiport Switch/1
  Navigation supervisor/2(Integrator Reset) -> Trajectory law - 2/4(Integrator Reset)
  formationOffset_m/1 -> Navigation supervisor/3(formationOffset_m), Trajectory law - 2/3(formationOffset_LS [m])
  iUASCom/1 -> Navigation supervisor/2(iUASCom), Launch law -1/2(iUASCom), Trajectory law - 2/2(iUASCom)
  Plant/1 -> Test signal generator - 3/1(Plant), Launch law -1/1(Plant), Trajectory law - 2/1(State), Navigation supervisor/1(Plant)
  Multiport Switch/1 -> CMD/1
  Trajectory law - 2/1(pc_NED_m) -> pc_NED_m/1
  Trajectory law - 2/2(vc_NED_mps) -> vc_NED_mps/1
  Test signal generator - 3/1(CMD) -> Multiport Switch/4
  Trim inputs - 4/1(u) -> Multiport Switch/5
  Trajectory law - 2/4(fstate_dx) -> fstate_dx/1
  fstate_dx_in/1 -> Trajectory law - 2/5(fstate_dx_in)

== system formationFlyingBlockset/Fixed wing avionics/Command laws/Subsystem ==
  In1 : Inport
  In2 : Inport  Port=2
  In3 : Inport  Port=3
  Action Port : ActionPort
  Visualize nominal NED position : formationFlyingBlockset/Visualize leader  mask_3dmodel=1
  wires:
  In3/1 -> Visualize nominal NED position/2
  In2/1 -> Visualize nominal NED position/1
  In1/1 -> Visualize nominal NED position/3

== system formationFlyingBlockset/Parrot drone open loop dynamics/Vehicle model/Parrot dynamics ==
  CMD : Inport  OutDataTypeStr=Bus: CMD_quadrotor
  EnvData : Inport  Port=2  OutDataTypeStr=Bus: Environment
  omega_bfrozen_rps : Inport  Port=3
  Vground_bfrozen_mps : Inport  Port=4
  eulers : Inport  Port=5
  Bus Selector : BusSelector  OutputSignals=cmd_engine_0t01
  Bus Selector3 : BusSelector  OutputSignals=a_mps,rho_kgm3,omegaw_bfrozen_rps,Vw_bfrozen_mps
  Bus Creator : BusCreator  Inputs=7
  Change rotation angle order : Selector  InputPortWidth=3  IndexOptions=Index vector (dialog)  Indices=[3 2 1]  OutputSizes=1
  Constant : Constant  Value=zeros(6,1)
  Constant2 : Constant  Value=0
  Constant3 : Constant  Value=0
  Derived aerodynamic conditions : uavsimBlockset_DerivedAerodynamicConditions/Derived aerodynamic conditions
  Modèle Force & Moment : Parrot_DCAS_lib/Modèle Force & Moment
  Mux : Mux  Inputs=2
  Quadcopter engine models : Parrot_DCAS_lib/Quadcopter engine models  SystemSampleTime=-1
  Scope{,1..3} (4 alike) : Scope
  Signal seems not to be used inside the block (what is vitesse_Rd supposed to mean anyway? : Ground
  "scale from normalized commands [0,1] to commanded angular rates [0, max]" : Gain  Gain=uavsim.parrot.omega_engine_max
  FMaero_bf : Outport
  AeroBus : Outport  Port=2  OutDataTypeStr=Bus: Aero
  Coefficients_windframe : Outport  Port=3
  wires:
  Bus Selector/1 -> "scale from normalized commands [0,1] to commanded angular rates [0, max]"/1  "<cmd_engine_0t01>"
  Bus Creator/1 -> AeroBus/1
  Derived aerodynamic conditions/6 -> Bus Creator/7  "qbar_Pa"
  Derived aerodynamic conditions/5 -> Bus Creator/6  "Ma"
  Derived aerodynamic conditions/3 -> Modèle Force & Moment/4, Bus Creator/5  "Va_mps"
  Derived aerodynamic conditions/2 -> Bus Creator/2  "beta_rad"
  Derived aerodynamic conditions/1 -> Bus Creator/1  "alpha_rad"
  Vground_bfrozen_mps/1 -> Scope3/1, Derived aerodynamic conditions/1
  Constant3/1 -> Bus Creator/4  "betaDot_rps"
  Constant2/1 -> Bus Creator/3  "alphaDot_rps"
  Bus Selector3/4 -> Derived aerodynamic conditions/5  "<Vw_bfrozen_mps>"
  Bus Selector3/3 -> Derived aerodynamic conditions/4  "<omegaw_bfrozen_rps>"
  Bus Selector3/2 -> Scope2/1, Derived aerodynamic conditions/3  "<rho_kgm3>"
  Bus Selector3/1 -> Scope1/1, Derived aerodynamic conditions/2  "<a_mps>"
  Constant/1 -> Coefficients_windframe/1
  Mux/1 -> FMaero_bf/1, Scope/1
  omega_bfrozen_rps/1 -> Modèle Force & Moment/3, Derived aerodynamic conditions/6
  EnvData/1 -> Bus Selector3/1
  Modèle Force & Moment/1 -> Mux/1
  Modèle Force & Moment/2 -> Mux/2
  Quadcopter engine models/1 -> Modèle Force & Moment/1
  "scale from normalized commands [0,1] to commanded angular rates [0, max]"/1 -> Quadcopter engine models/1
  eulers/1 -> Change rotation angle order/1
  Change rotation angle order/1 -> Modèle Force & Moment/2
  Signal seems not to be used inside the block (what is vitesse_Rd supposed to mean anyway?/1 -> Modèle Force & Moment/5
  CMD/1 -> Bus Selector/1
